simulink subsystem "FCS_Outputs"  (R2025a)
settings: Solver=VariableStepAuto  StartTime=0.0  StopTime=10.0  RelTol=1e-3
settings Model: Creator=gurt1  LastModifiedBy=gurt1

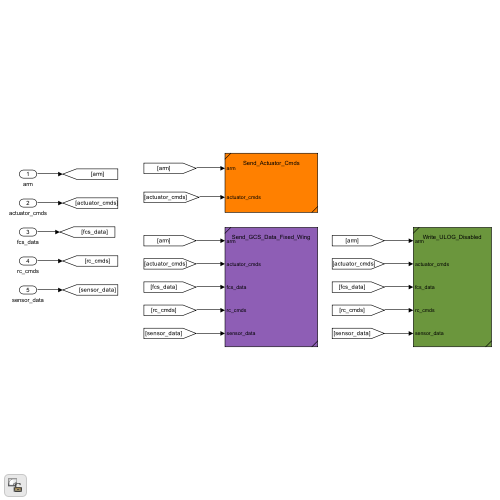
[thumbnail: Simulink's stored preview of the top-level diagram]
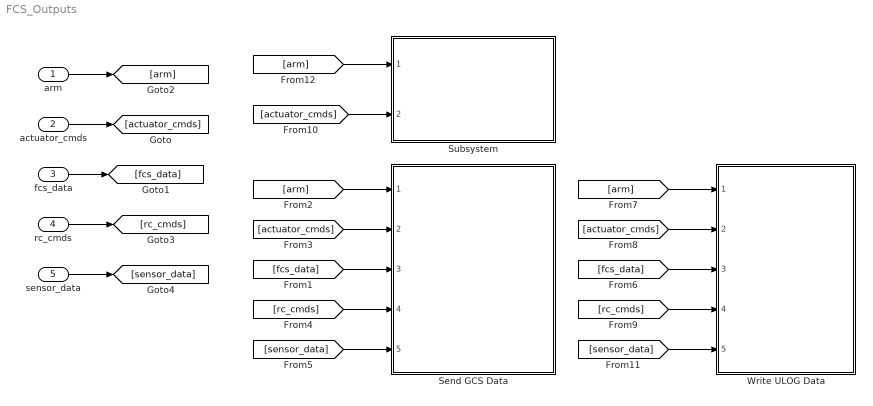
== system FCS_Outputs ==
  arm : Inport
  actuator_cmds : Inport  Port=2
  fcs_data : Inport  Port=3
  rc_cmds : Inport  Port=4
  sensor_data : Inport  Port=5
  Send GCS Data : Subsystem  ReferencedSubsystem=Send_GCS_Data
  Subsystem : Subsystem  ReferencedSubsystem=Send_Actuator_Cmds
  Write ULOG Data : Subsystem  ReferencedSubsystem=Write_ULOG_Disabled
  wires:
  actuator_cmds/1 -> [actuator_cmds]
  fcs_data/1 -> [fcs_data]
  arm/1 -> [arm]
  rc_cmds/1 -> [rc_cmds]
  sensor_data/1 -> [sensor_data]
  [arm] -> Write ULOG Data/1
  [actuator_cmds] -> Write ULOG Data/2
  [fcs_data] -> Write ULOG Data/3
  [rc_cmds] -> Write ULOG Data/4
  [sensor_data] -> Write ULOG Data/5
  [arm] -> Send GCS Data/1
  [actuator_cmds] -> Send GCS Data/2
  [fcs_data] -> Send GCS Data/3
  [rc_cmds] -> Send GCS Data/4
  [sensor_data] -> Send GCS Data/5
  [arm] -> Subsystem/1
  [actuator_cmds] -> Subsystem/2
